simulink model "sst_cllc_ttype_inv"  (R2026a)
settings: Solver=ode23tb  StopTime=simlength  FixedStep=tc  MaxStep=glb_time.tc
values from neighbouring files (symbols this model uses):
  afe_ctrl = ctrl_afe_setup(glb_time.ts_afe, grid_emu.omega_grid_nom)    [init_model.m]
  cllc_ctrl = ctrl_cllc_setup(kp_udc, ki_udc, kp_idc, ki_idc)    [init_model.m]
  glb_time = timing_setup(fpwm_afe, trgo_afe, fpwm_inv, trgo_inv, fpwm_single_phase_inv, trgo_single_phase_inv, fpwm_dab, trgo_dab,      fpwm_psfbc, trgo_psfbc, fpwm_isop_rail, trgo_isop_rail, fpwm_cllc, trgo_cllc, t_measure, tc_factor, tc_decimation, delay_pwm, dead_time_afe,      dead_time_inv, dead_time_single_phase_inv, dead_time_dab, dead_time_psfbc, dead_time_isop_rail, dead_time_cllc)    [init_model.m]
  grid_emu = grid_three_phase_emulator('Dyn11', delta_star, grid_nominal_power, application_voltage, us1, us2, fgrid,                  eq_grid_inductance, eq_grid_resistance, eta, ucc, i1m, p_iron, n1, n2, core_area, core_length, mur,                  up_xi_pu_ref, up_eta_pu_ref, un_xi_pu_ref, un_eta_pu_ref)    [init_model.m]
  lithium_ion_battery_1 = lithium_ion_battery_setup(nominal_battery_voltage_1, nominal_battery_power, initial_battery_soc, glb_time.ts_dab)    [init_model.m]
  omega_set = frequency_set*2*pi    (= 1884.95559215)    [init_model.m]
  single_phase_inverter_ctrl = ctrl_single_phase_inverter_setup(glb_time.ts_inv, pres_ctrl.omega_set,      dqvector_pi.kp_inv, dqvector_pi.ki_inv, pres_ctrl.kp_rpi, pres_ctrl.ki_rpi, pres_ctrl.delta_rpi)    [init_model.m]
  sst_num_of_modules = 2    [init_model.m]
undefined symbols (not defined in the file or in its folder): hwdata
libraries: fl_lib x62, nesl_utility x38, discrete_time_low_pass_filter x8, full_bridge_ideal_switch x4, full_bridge_mosfet_based_with_thermal_model x4, full_bridge_mosfet_based_with_thermal_model_zvs x4, lithium_ion_battery x2, single_phase_transformer x2, dab_single_phase_pwm_modulator x2, dclink_for_three_levels x2, full_bridge_three_level_ttype_ideal_switch_based_model x2, full_bridge_three_level_ttype_mosfet_based_model x2
(part 2 of 5)

== system sst_cllc_ttype_inv/global timing/time_cllc_A ==
  correction_time : Inport
  Constant : Constant
  Gain : Gain  Gain=k
  Product : Product
  Sum : Sum  Inputs=|++
  time_1 : Clock
  Out1 : Outport
  wires:
  time_1/1 -> Gain/1
  Gain/1 -> Product/1
  Product/1 -> Out1/1
  correction_time/1 -> Sum/1
  Constant/1 -> Sum/2
  Sum/1 -> Product/2

== system sst_cllc_ttype_inv/global timing/time_cllc_B ==
  correction_time : Inport
  Constant : Constant
  Gain : Gain  Gain=k
  Product : Product
  Sum : Sum  Inputs=|++
  time_1 : Clock
  Out1 : Outport
  wires:
  time_1/1 -> Gain/1
  Gain/1 -> Product/1
  Product/1 -> Out1/1
  correction_time/1 -> Sum/1
  Constant/1 -> Sum/2
  Sum/1 -> Product/2

== system sst_cllc_ttype_inv/global timing/time_master ==
  Gain : Gain  Gain=k
  time_1 : Clock
  Out1 : Outport
  wires:
  Gain/1 -> Out1/1
  time_1/1 -> Gain/1

== system sst_cllc_ttype_inv/line_source/phase_gen ==
  Constant4 : Constant  Value=grid_emu.omega_grid_nom
  Integrator : Integrator
  bounder1 : MATLAB Function  TreatAsAtomicUnit=on
  phase_gen : Outport  VectorParamsAs1DForOutWhenUnconnected=off
  wires:
  Constant4/1 -> Integrator/1
  Integrator/1 -> bounder1/1(u)
  bounder1/1(y) -> phase_gen/1  "grid_emu_phase"

== system sst_cllc_ttype_inv/scopes/scopes_dcdc_modA ==
  Bus Selector : BusSelector  OutputSignals=mosfet_ploss_Q1,mosfet_ploss_Q2
  Bus Selector1 : BusSelector  OutputSignals=mosfet_ploss_Q1,mosfet_ploss_Q2
  cllc TR i2/i1 modA : Scope  NumInputPorts=2
      settings: ActiveDisplayYMinimum=-1515.8601129634949  ActiveDisplayYMaximum=1519.4045908602914  DataLoggingVariableName=ScopeData13
  cllc TR u2/u1 modA : Scope  NumInputPorts=2
      settings: ActiveDisplayYMinimum=-893.62031856834165  ActiveDisplayYMaximum=653.92363611228757  DataLoggingVariableName=ScopeData4
  cllc current output/input modA : Scope  NumInputPorts=2
      settings: ActiveDisplayYMinimum=-34.407086049322743  ActiveDisplayYMaximum=284.20809963586862  DataLoggingVariableName=ScopeData8
  cllc voltage input/output modA : Scope  NumInputPorts=2
      settings: ActiveDisplayYMinimum=-224.45374462345234  ActiveDisplayYMaximum=1977.0471198962268  DataLoggingVariableName=ScopeData10
  cllc_analysis_modA : Scope  NumInputPorts=4
      settings: ActiveDisplayYMinimum=-29.182723661894556  ActiveDisplayYMaximum=23.685544723854832  DataLoggingVariableName=ScopeData15
  cllc_analysis_power loss : Scope  NumInputPorts=4
      settings: ActiveDisplayYMinimum=17.348303631345402  ActiveDisplayYMaximum=238.28763733532384  DataLoggingVariableName=ScopeData17
  dab outputs modA : Scope  NumInputPorts=2
      settings: ActiveDisplayYMinimum=-691.31278967103344  ActiveDisplayYMaximum=557.00399497186572  DataLoggingVariableName=ScopeData6
  wires:
  [cllc_voltage_input_modA] -> cllc voltage input/output modA/1  "cllc_voltage_input_modA"
  [cllc_current_output_modA] -> cllc current output/input modA/1  "cllc_current_output_modA"
  [cllc_voltage_output_modA] -> cllc voltage input/output modA/2  "cllc_voltage_output_modA"
  [cllc_current_input_modA] -> cllc current output/input modA/2  "cllc_current_input_modA"
  [i2_cllc_transformer_modA] -> cllc TR i2/i1 modA/1  "i2_cllc_transformer_modA"
  [i1_cllc_transformer_modA] -> cllc TR i2/i1 modA/2  "i1_cllc_transformer_modA"
  [u2_cllc_transformer_modA] -> cllc TR u2/u1 modA/1  "u2_cllc_transformer_modA"
  [u1_cllc_transformer_modA] -> cllc TR u2/u1 modA/2  "u1_cllc_transformer_modA"
  [cllc_voltage_output_modA] -> dab outputs modA/2  "cllc_voltage_output_modA"
  [cllc_current_output_modA] -> dab outputs modA/1  "cllc_current_output_modA"
  [i2_cllc_transformer_modA] -> cllc_analysis_modA/1  "i2_cllc_transformer_modA"
  [i1_cllc_transformer_modA] -> cllc_analysis_modA/2  "i1_cllc_transformer_modA"
  [u1_cllc_transformer_modA] -> cllc_analysis_modA/3  "u1_cllc_transformer_modA"
  [u2_cllc_transformer_modA] -> cllc_analysis_modA/4  "u2_cllc_transformer_modA"
  [inverter_1_cllc_mosfet_zvs_modA] -> Bus Selector/1
  [inverter_2_cllc_mosfet_zvs_modA] -> Bus Selector1/1
  Bus Selector/1 -> cllc_analysis_power loss/1  "<mosfet_ploss_Q1>"
  Bus Selector/2 -> cllc_analysis_power loss/2  "<mosfet_ploss_Q2>"
  Bus Selector1/1 -> cllc_analysis_power loss/3  "<mosfet_ploss_Q1>"
  Bus Selector1/2 -> cllc_analysis_power loss/4  "<mosfet_ploss_Q2>"

== system sst_cllc_ttype_inv/scopes/scopes_dcdc_modB ==
  cllc TR i2/i1 modB : Scope  NumInputPorts=2
      settings: ActiveDisplayYMinimum=-700.08630880673149  ActiveDisplayYMaximum=469.74027472719069  DataLoggingVariableName=ScopeData13
  cllc TR u2/u1 modB : Scope  NumInputPorts=2
      settings: ActiveDisplayYMinimum=-893.62031856834165  ActiveDisplayYMaximum=653.92363611228757  DataLoggingVariableName=ScopeData4
  cllc current output/input modB : Scope  NumInputPorts=2
      settings: ActiveDisplayYMinimum=-7335.7913745283768  ActiveDisplayYMaximum=23819.434208451414  DataLoggingVariableName=ScopeData8
  cllc outputs modB : Scope  NumInputPorts=2
      settings: ActiveDisplayYMinimum=-1276.7812228163118  ActiveDisplayYMaximum=1202.3221787513703  DataLoggingVariableName=ScopeData6
  cllc voltage input/output modB : Scope  NumInputPorts=2
      settings: ActiveDisplayYMinimum=-237.60937353263552  ActiveDisplayYMaximum=2138.4843617937204  DataLoggingVariableName=ScopeData10
  cllc_analysis_modB : Scope  NumInputPorts=4
      settings: ActiveDisplayYMinimum=-1515.8601129634949  ActiveDisplayYMaximum=1519.4045908602914  DataLoggingVariableName=ScopeData15
  wires:
  [u2_cllc_transformer_modB] -> cllc_analysis_modB/4  "u2_cllc_transformer_modB"
  [u1_cllc_transformer_modB] -> cllc_analysis_modB/3  "u1_cllc_transformer_modB"
  [i1_cllc_transformer_modB] -> cllc_analysis_modB/2  "i1_cllc_transformer_modB"
  [i2_cllc_transformer_modB] -> cllc_analysis_modB/1  "i2_cllc_transformer_modB"
  [cllc_current_output_modB] -> cllc outputs modB/1  "cllc_current_output_modB"
  [cllc_voltage_output_modB] -> cllc outputs modB/2  "cllc_voltage_output_modB"
  [u1_cllc_transformer_modB] -> cllc TR u2/u1 modB/2  "u1_cllc_transformer_modB"
  [u2_cllc_transformer_modB] -> cllc TR u2/u1 modB/1  "u2_cllc_transformer_modB"
  [i1_cllc_transformer_modB] -> cllc TR i2/i1 modB/2  "i1_cllcb_transformer_modB"
  [i2_cllc_transformer_modB] -> cllc TR i2/i1 modB/1  "i2_cllc_transformer_modB"
  [cllc_current_input_modB] -> cllc current output/input modB/2  "cllc_current_input_modB"
  [cllc_voltage_output_modB] -> cllc voltage input/output modB/2  "cllc_voltage_output_modB"
  [cllc_current_output_modB] -> cllc current output/input modB/1  "cllc_current_output_modB"
  [cllc_voltage_input_modB] -> cllc voltage input/output modB/1  "cllc_voltage_input_modB"

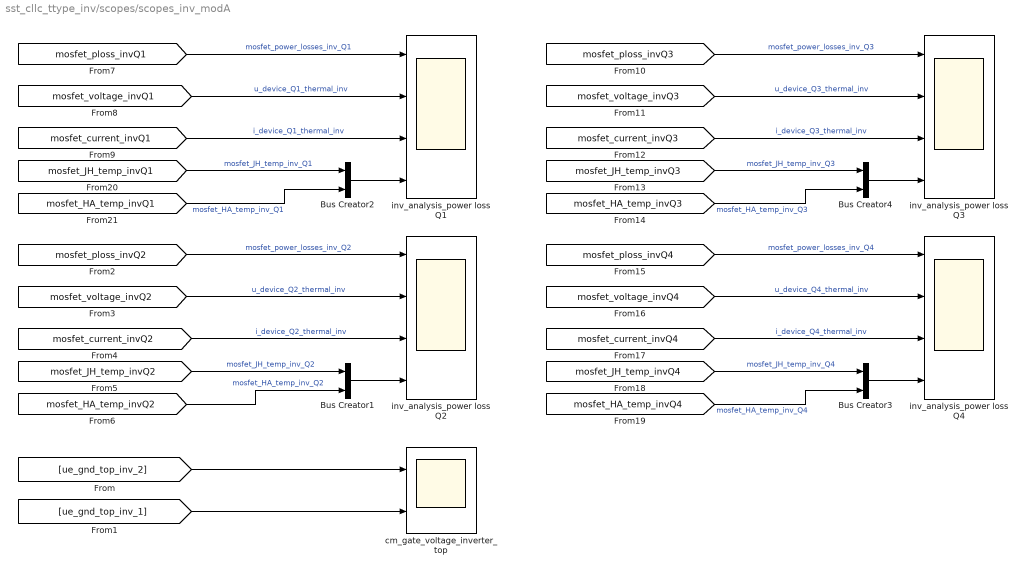
== system sst_cllc_ttype_inv/scopes/scopes_inv_modA ==
  Bus Creator{1..4} (4 alike) : BusCreator  Inputs=2
  cm_gate_voltage_inverter_top : Scope  NumInputPorts=2
      settings: ActiveDisplayYMinimum=-1089.6954299405313  ActiveDisplayYMaximum=1165.8713445946826  DataLoggingVariableName=ScopeData22
  inv_analysis_power loss Q{1..4} (4 alike) : Scope  NumInputPorts=4
      inv_analysis_power loss Q1 settings: ActiveDisplayYMinimum=252.03887543128099  ActiveDisplayYMaximum=654.5130246681365  DataLoggingVariableName=ScopeData18
      inv_analysis_power loss Q2 settings: ActiveDisplayYMinimum=1215.5585157804567  ActiveDisplayYMaximum=1882.3509853926439  DataLoggingVariableName=ScopeData5
      inv_analysis_power loss Q3 settings: ActiveDisplayYMinimum=1399.7218598743666  ActiveDisplayYMaximum=1614.3940109339064  DataLoggingVariableName=ScopeData16
      inv_analysis_power loss Q4 settings: ActiveDisplayYMinimum=401.80036733196005  ActiveDisplayYMaximum=489.90080295034829  DataLoggingVariableName=ScopeData19
  wires:
  [mosfet_JH_temp_invQ1] -> Bus Creator2/1  "mosfet_JH_temp_inv_Q1"
  [mosfet_voltage_invQ1] -> inv_analysis_power loss Q1/2  "u_device_Q1_thermal_inv"
  [mosfet_current_invQ1] -> inv_analysis_power loss Q1/3  "i_device_Q1_thermal_inv"
  [mosfet_HA_temp_invQ1] -> Bus Creator2/2  "mosfet_HA_temp_inv_Q1"
  Bus Creator2/1 -> inv_analysis_power loss Q1/4
  [mosfet_ploss_invQ1] -> inv_analysis_power loss Q1/1  "mosfet_power_losses_inv_Q1"
  [ue_gnd_top_inv_2] -> cm_gate_voltage_inverter_top/1
  [ue_gnd_top_inv_1] -> cm_gate_voltage_inverter_top/2
  [mosfet_ploss_invQ2] -> inv_analysis_power loss Q2/1  "mosfet_power_losses_inv_Q2"
  Bus Creator1/1 -> inv_analysis_power loss Q2/4
  [mosfet_HA_temp_invQ2] -> Bus Creator1/2  "mosfet_HA_temp_inv_Q2"
  [mosfet_current_invQ2] -> inv_analysis_power loss Q2/3  "i_device_Q2_thermal_inv"
  [mosfet_voltage_invQ2] -> inv_analysis_power loss Q2/2  "u_device_Q2_thermal_inv"
  [mosfet_JH_temp_invQ2] -> Bus Creator1/1  "mosfet_JH_temp_inv_Q2"
  [mosfet_JH_temp_invQ4] -> Bus Creator3/1  "mosfet_JH_temp_inv_Q4"
  [mosfet_voltage_invQ4] -> inv_analysis_power loss Q4/2  "u_device_Q4_thermal_inv"
  [mosfet_current_invQ4] -> inv_analysis_power loss Q4/3  "i_device_Q4_thermal_inv"
  [mosfet_HA_temp_invQ4] -> Bus Creator3/2  "mosfet_HA_temp_inv_Q4"
  Bus Creator3/1 -> inv_analysis_power loss Q4/4
  [mosfet_ploss_invQ4] -> inv_analysis_power loss Q4/1  "mosfet_power_losses_inv_Q4"
  [mosfet_ploss_invQ3] -> inv_analysis_power loss Q3/1  "mosfet_power_losses_inv_Q3"
  Bus Creator4/1 -> inv_analysis_power loss Q3/4
  [mosfet_HA_temp_invQ3] -> Bus Creator4/2  "mosfet_HA_temp_inv_Q3"
  [mosfet_current_invQ3] -> inv_analysis_power loss Q3/3  "i_device_Q3_thermal_inv"
  [mosfet_voltage_invQ3] -> inv_analysis_power loss Q3/2  "u_device_Q3_thermal_inv"
  [mosfet_JH_temp_invQ3] -> Bus Creator4/1  "mosfet_JH_temp_inv_Q3"

== system sst_cllc_ttype_inv/scopes/scopes_inv_modB ==
  cm_gate_voltage_inverter_bottom : Scope  NumInputPorts=2
      settings: ActiveDisplayYMinimum=-1241.6958905586757  ActiveDisplayYMaximum=1224.9152234663466  DataLoggingVariableName=ScopeData22
  device_voltage_current_inv Q1 modB : Scope  NumInputPorts=3
      settings: ActiveDisplayYMinimum=-119.06518095025848  ActiveDisplayYMaximum=1054.0032225267662  DataLoggingVariableName=ScopeData20
  wires:
  [ue_gnd_bottom_inv_1] -> cm_gate_voltage_inverter_bottom/2
  [ue_gnd_bottom_inv_2] -> cm_gate_voltage_inverter_bottom/1
  [i_device_Q1_ideal_inv_modB] -> device_voltage_current_inv Q1 modB/2  "iQ1"
  [u_device_Q1_ideal_inv_modB] -> device_voltage_current_inv Q1 modB/1  "uQ1"
  [udc12_inverter_modB] -> device_voltage_current_inv Q1 modB/3  "udcs"

== system sst_cllc_ttype_inv/single_phase_inverter_modA/dclink ==
  Open Circuit : fl_lib/Electrical/Electrical Elements/Open Circuit  v_specify=off  v_priority=None  v=0 V  v_nominal_specify=off  v_nominal_value=1  v_nominal_unit=V
  dclink : dclink_for_three_levels/dclink  Cdc1_m=hwdata.single_phase_inverter.CFi1  Cdc2_m=hwdata.single_phase_inverter.CFi2  Rudc_measure=107e3  Vdc_scale=hwdata.cllc.udc2_bez  Vdc1_m_init=hwdata.cllc.udc2_bez/2  Vdc2_m_init=hwdata.cllc.udc2_bez/2
  references : Subsystem
  Udc(+) : PMIOPort  Side=Right
  np : PMIOPort  Port=2  Side=Right
  Udc(-) : PMIOPort  Port=3  Side=Right
  udc(+) : PMIOPort  Port=4  Side=Left
  udc(-) : PMIOPort  Port=5  Side=Left
  wires:
  dclink/1 -> references/1(m)
  connections:
  Open Circuit/LConn1 -- dclink/RConn2
  udc(+)/RConn1 -- dclink/RConn1
  udc(-)/RConn1 -- dclink/RConn3
  Udc(+)/RConn1 -- dclink/LConn1
  Udc(-)/RConn1 -- dclink/LConn3
  dclink/LConn2 -- np/RConn1

== system sst_cllc_ttype_inv/single_phase_inverter_modA/output_filter ==
  Capacitor : fl_lib/Electrical/Electrical Elements/Capacitor  c=hwdata.single_phase_inverter.CFu F  r=hwdata.single_phase_inverter.RCFu Ohm  g=0 1/Ohm  i_specify=off  i_priority=None  i=0 A  i_nominal_specify=off  i_nominal_value=1  i_nominal_unit=A  v_specify=off  v_priority=None  v=0 V  v_nominal_specify=off  v_nominal_value=1  v_nominal_unit=V  vc_specify=off  vc_priority=High  vc=0 V  vc_nominal_specify=off  vc_nominal_value=1  vc_nominal_unit=V
  Current Sensor : fl_lib/Electrical/Electrical Sensors/Current Sensor
  Current Sensor1 : fl_lib/Electrical/Electrical Sensors/Current Sensor
  LFu1 : fl_lib/Electrical/Electrical Elements/Inductor  l=hwdata.single_phase_inverter.LFu1 H  r=hwdata.single_phase_inverter.RLFu1 Ohm  g=1e-9 1/Ohm  i_specify=off  i_priority=None  i=0 A  i_nominal_specify=off  i_nominal_value=1  i_nominal_unit=A  v_specify=off  v_priority=None  v=0 V  v_nominal_specify=off  v_nominal_value=1  v_nominal_unit=V  i_L_specify=off  i_L_priority=High  i_L=0 A  i_L_nominal_specify=off  i_L_nominal_value=1  i_L_nominal_unit=A
  LFu2 : fl_lib/Electrical/Electrical Elements/Inductor  l=hwdata.single_phase_inverter.LFu2 H  r=hwdata.single_phase_inverter.RLFu2 Ohm  g=1e-9 1/Ohm  i_specify=off  i_priority=None  i=0 A  i_nominal_specify=off  i_nominal_value=1  i_nominal_unit=A  v_specify=off  v_priority=None  v=0 V  v_nominal_specify=off  v_nominal_value=1  v_nominal_unit=V  i_L_specify=off  i_L_priority=High  i_L=0 A  i_L_nominal_specify=off  i_L_nominal_value=1  i_L_nominal_unit=A
  Voltage Sensor1 : fl_lib/Electrical/Electrical Sensors/Voltage Sensor
  Voltage Sensor2 : fl_lib/Electrical/Electrical Sensors/Voltage Sensor
  iph : nesl_utility/PS-Simulink Converter  PhysicalDomain=network_engine_domain  SubClassName=ps_output  LeftPortType=input  RightPortType=output  PseudoPeriodic=off  Frequencies=[]  VectorFormat=1-D array  Unit=A  AffineConversion=off
  iph1 : nesl_utility/PS-Simulink Converter  PhysicalDomain=network_engine_domain  SubClassName=ps_output  LeftPortType=input  RightPortType=output  PseudoPeriodic=off  Frequencies=[]  VectorFormat=1-D array  Unit=A  AffineConversion=off
  uph1 : nesl_utility/PS-Simulink Converter  PhysicalDomain=network_engine_domain  SubClassName=ps_output  LeftPortType=input  RightPortType=output  PseudoPeriodic=off  Frequencies=[]  VectorFormat=1-D array  Unit=V  AffineConversion=off
  uph2 : nesl_utility/PS-Simulink Converter  PhysicalDomain=network_engine_domain  SubClassName=ps_output  LeftPortType=input  RightPortType=output  PseudoPeriodic=off  Frequencies=[]  VectorFormat=1-D array  Unit=V  AffineConversion=off
  Uac(+) : PMIOPort  Side=Left
  uac(+) : PMIOPort  Port=2  Side=Right
  Uac(-) : PMIOPort  Port=3  Side=Left
  uac(-) : PMIOPort  Port=4  Side=Right
  tag scope: afe_current_output_modA=global, afe_is_modA=global, afe_us_modA=global, afe_voltage_output_modA=global
  wires:
  uph1/1 -> [afe_voltage_output_modA]  "inverter_voltage_output"
  iph/1 -> [afe_current_output_modA]  "inverter_current_output"
  iph1/1 -> [afe_is_modA]  "inverter_is_modA"
  uph2/1 -> [afe_us_modA]  "inverter_us_modA"
  connections:
  Voltage Sensor2/LConn1 -- Current Sensor1/RConn2 -- LFu1/LConn1
  Current Sensor/RConn2 -- uac(+)/RConn1 -- Voltage Sensor1/LConn1
  Voltage Sensor1/RConn2 -- Capacitor/RConn1 -- LFu2/RConn1 -- uac(-)/RConn1
  iph/LConn1 -- Current Sensor/RConn1
  Voltage Sensor1/RConn1 -- uph1/LConn1
  LFu1/RConn1 -- Capacitor/LConn1 -- Current Sensor/LConn1
  Uac(-)/RConn1 -- Voltage Sensor2/RConn2 -- LFu2/LConn1
  iph1/LConn1 -- Current Sensor1/RConn1
  Voltage Sensor2/RConn1 -- uph2/LConn1
  Uac(+)/RConn1 -- Current Sensor1/LConn1

== system sst_cllc_ttype_inv/single_phase_inverter_modA/single phase afe ==
  gate_commands : Inport
  ideal_switch_based_three_level_inverter_ttype : full_bridge_three_level_ttype_ideal_switch_based_model/ideal_switch_based_three_level_inverter_ttype  Commented=on  Vth=ideal_switch.Vth  Ron=ideal_switch.Rds_on  Vdon_diode=ideal_switch.Vdon_diode  Rdon_diode=ideal_switch.Rdon_diode  Csnubber=ideal_switch.Csnubber  Rsnubber=ideal_switch.Rsnubber
  mosfet_based_three_level_inverter_ttype : full_bridge_three_level_ttype_mosfet_based_model/mosfet_based_three_level_inverter_ttype  Vth_m=mosfet.inv.Vth  Rds_on_m=mosfet.inv.Rds_on  Eon_m=mosfet.inv.Eon  Eoff_m=mosfet.inv.Eoff  Erec_m=mosfet.inv.Err  Ion_sw_loss_m=mosfet.inv.Ion_sw_losses  Voff_sw_loss_m=mosfet.inv.Voff_sw_losses  Vdon_diode_m=mosfet.inv.Vdon_diode  Rdon_diode_m=mosfet.inv.Rdon_diode  rth_mosfet_JH_m=mosfet.inv.Rth_mosfet_JH  rth_mosfet_HA_m=heatsink.Rth_mosfet_HA  Csnubber_m=mosfet.inv.Csnubber  Rsnubber_m=mosfet.inv.Rsnubber  JunctionTermalMass_m=mosfet.inv.JunctionTermalMass  mass_heatsink_m=heatsink.no_weight  specific_heat_m=heatsink.cp  Tambient_m=heatsink.Tambient  DThs_init_m=heatsink.DThs_init  tc_m=glb_time.tc
  references : Subsystem
  uac_out(+) : PMIOPort  Side=Left
  uac_out(-) : PMIOPort  Port=2  Side=Left
  udc(+) : PMIOPort  Port=3  Side=Right
  np : PMIOPort  Port=4  Side=Right
  udc(-) : PMIOPort  Port=5  Side=Right
  wires:
  gate_commands/1 -> mosfet_based_three_level_inverter_ttype/1, ideal_switch_based_three_level_inverter_ttype/1
  mosfet_based_three_level_inverter_ttype/1 -> references/1(m)
  connections:
  ideal_switch_based_three_level_inverter_ttype/LConn2 -- mosfet_based_three_level_inverter_ttype/LConn2 -- uac_out(-)/RConn1
  ideal_switch_based_three_level_inverter_ttype/RConn1 -- mosfet_based_three_level_inverter_ttype/RConn1 -- udc(+)/RConn1
  ideal_switch_based_three_level_inverter_ttype/LConn1 -- mosfet_based_three_level_inverter_ttype/LConn1 -- uac_out(+)/RConn1
  ideal_switch_based_three_level_inverter_ttype/RConn3 -- mosfet_based_three_level_inverter_ttype/RConn3 -- udc(-)/RConn1
  ideal_switch_based_three_level_inverter_ttype/RConn2 -- mosfet_based_three_level_inverter_ttype/RConn2 -- np/RConn1

== system sst_cllc_ttype_inv/single_phase_inverter_modA/single phase inverter control ==
  acquisition_and_scaling_current : Subsystem  Commented=on
  acquisition_and_scaling_current_with_white_noise : Subsystem
  acquisition_and_scaling_dc_voltage : Subsystem
  acquisition_and_scaling_grid_voltage_ac : Subsystem
  acquisition_and_scaling_voltage : Subsystem
  inverter_current_output_pu_reference : Subsystem
  pwm modulator : Subsystem
  single_phase_inverter_ctrl : Subsystem
  gate_cmds : Outport
  tag scope: afe_phase_grid_hat_modA=global, udq_ctrl_out_modA=global
  wires:
  [afe_is_modA] -> acquisition_and_scaling_current_with_white_noise/1(in)
  pwm modulator/1(gate_cmds) -> gate_cmds/1
  [TRGO_AFE_modA] -> single_phase_inverter_ctrl/Trigger
  [afe_voltage_output_modA] -> acquisition_and_scaling_voltage/1(in)
  single_phase_inverter_ctrl/1(u_ctrl_out) -> pwm modulator/1(vout)
  acquisition_and_scaling_current_with_white_noise/1(out) -> single_phase_inverter_ctrl/2(afe_current_output_pu)  "afe_current_output_pu"
  acquisition_and_scaling_voltage/1(out) -> single_phase_inverter_ctrl/1(afe_voltage_output_pu)  "afe_voltage_output_pu"
  inverter_current_output_pu_reference/1(afe_current_output_pu_reference) -> single_phase_inverter_ctrl/3(afe_current output_pu_reference)  "afe_current_output_pu_reference"
  [dclink_voltage_modA] -> acquisition_and_scaling_dc_voltage/1(in)
  acquisition_and_scaling_dc_voltage/1(out) -> single_phase_inverter_ctrl/4(dclink_voltage_pu)  "dclink_voltage_pu"
  [time_afe_module_A] -> single_phase_inverter_ctrl/5(local_time)
  [ac_grid_voltage] -> acquisition_and_scaling_grid_voltage_ac/1(in)
  acquisition_and_scaling_grid_voltage_ac/1(out) -> single_phase_inverter_ctrl/6(ugrid_pu)  "ug_abc"
  single_phase_inverter_ctrl/2(phase_grid_hat) -> [afe_phase_grid_hat_modA]
  single_phase_inverter_ctrl/3(udq_ctrl_out) -> [udq_ctrl_out_modA]

== system sst_cllc_ttype_inv/single_phase_inverter_modB/dclink ==
  Open Circuit : fl_lib/Electrical/Electrical Elements/Open Circuit  v_specify=off  v_priority=None  v=0 V  v_nominal_specify=off  v_nominal_value=1  v_nominal_unit=V
  dclink : dclink_for_three_levels/dclink  Cdc1_m=hwdata.single_phase_inverter.CFi1  Cdc2_m=hwdata.single_phase_inverter.CFi2  Rudc_measure=107e3  Vdc_scale=hwdata.cllc.udc2_bez  Vdc1_m_init=hwdata.cllc.udc2_bez/2  Vdc2_m_init=hwdata.cllc.udc2_bez/2
  references : Subsystem
  Udc(+) : PMIOPort  Side=Right
  np : PMIOPort  Port=2  Side=Right
  Udc(-) : PMIOPort  Port=3  Side=Right
  udc(+) : PMIOPort  Port=4  Side=Left
  udc(-) : PMIOPort  Port=5  Side=Left
  wires:
  dclink/1 -> references/1(m)
  connections:
  dclink/LConn2 -- np/RConn1
  Udc(-)/RConn1 -- dclink/LConn3
  Udc(+)/RConn1 -- dclink/LConn1
  udc(-)/RConn1 -- dclink/RConn3
  udc(+)/RConn1 -- dclink/RConn1
  Open Circuit/LConn1 -- dclink/RConn2

== system sst_cllc_ttype_inv/single_phase_inverter_modB/output_filter ==
  Capacitor : fl_lib/Electrical/Electrical Elements/Capacitor  c=hwdata.single_phase_inverter.CFu F  r=hwdata.single_phase_inverter.RCFu Ohm  g=0 1/Ohm  i_specify=off  i_priority=None  i=0 A  i_nominal_specify=off  i_nominal_value=1  i_nominal_unit=A  v_specify=off  v_priority=None  v=0 V  v_nominal_specify=off  v_nominal_value=1  v_nominal_unit=V  vc_specify=off  vc_priority=High  vc=0 V  vc_nominal_specify=off  vc_nominal_value=1  vc_nominal_unit=V
  Current Sensor : fl_lib/Electrical/Electrical Sensors/Current Sensor
  Current Sensor1 : fl_lib/Electrical/Electrical Sensors/Current Sensor
  LFu1 : fl_lib/Electrical/Electrical Elements/Inductor  l=hwdata.single_phase_inverter.LFu1 H  r=hwdata.single_phase_inverter.RLFu1 Ohm  g=1e-9 1/Ohm  i_specify=off  i_priority=None  i=0 A  i_nominal_specify=off  i_nominal_value=1  i_nominal_unit=A  v_specify=off  v_priority=None  v=0 V  v_nominal_specify=off  v_nominal_value=1  v_nominal_unit=V  i_L_specify=off  i_L_priority=High  i_L=0 A  i_L_nominal_specify=off  i_L_nominal_value=1  i_L_nominal_unit=A
  LFu2 : fl_lib/Electrical/Electrical Elements/Inductor  l=hwdata.single_phase_inverter.LFu2 H  r=hwdata.single_phase_inverter.RLFu2 Ohm  g=1e-9 1/Ohm  i_specify=off  i_priority=None  i=0 A  i_nominal_specify=off  i_nominal_value=1  i_nominal_unit=A  v_specify=off  v_priority=None  v=0 V  v_nominal_specify=off  v_nominal_value=1  v_nominal_unit=V  i_L_specify=off  i_L_priority=High  i_L=0 A  i_L_nominal_specify=off  i_L_nominal_value=1  i_L_nominal_unit=A
  Voltage Sensor1 : fl_lib/Electrical/Electrical Sensors/Voltage Sensor
  Voltage Sensor2 : fl_lib/Electrical/Electrical Sensors/Voltage Sensor
  iph : nesl_utility/PS-Simulink Converter  PhysicalDomain=network_engine_domain  SubClassName=ps_output  LeftPortType=input  RightPortType=output  PseudoPeriodic=off  Frequencies=[]  VectorFormat=1-D array  Unit=A  AffineConversion=off
  iph1 : nesl_utility/PS-Simulink Converter  PhysicalDomain=network_engine_domain  SubClassName=ps_output  LeftPortType=input  RightPortType=output  PseudoPeriodic=off  Frequencies=[]  VectorFormat=1-D array  Unit=A  AffineConversion=off
  uph1 : nesl_utility/PS-Simulink Converter  PhysicalDomain=network_engine_domain  SubClassName=ps_output  LeftPortType=input  RightPortType=output  PseudoPeriodic=off  Frequencies=[]  VectorFormat=1-D array  Unit=V  AffineConversion=off
  uph2 : nesl_utility/PS-Simulink Converter  PhysicalDomain=network_engine_domain  SubClassName=ps_output  LeftPortType=input  RightPortType=output  PseudoPeriodic=off  Frequencies=[]  VectorFormat=1-D array  Unit=V  AffineConversion=off
  Uac(+) : PMIOPort  Side=Left
  uac(+) : PMIOPort  Port=2  Side=Right
  Uac(-) : PMIOPort  Port=3  Side=Left
  uac(-) : PMIOPort  Port=4  Side=Right
  tag scope: afe_current_output_modB=global, afe_is_modB=global, afe_us_modB=global, afe_voltage_output_modB=global
  wires:
  uph2/1 -> [afe_us_modB]  "inverter_us_modA"
  iph1/1 -> [afe_is_modB]  "inverter_is_modA"
  iph/1 -> [afe_current_output_modB]  "inverter_current_output"
  uph1/1 -> [afe_voltage_output_modB]  "inverter_voltage_output"
  connections:
  Uac(+)/RConn1 -- Current Sensor1/LConn1
  Voltage Sensor2/RConn1 -- uph2/LConn1
  iph1/LConn1 -- Current Sensor1/RConn1
  LFu2/LConn1 -- Voltage Sensor2/RConn2 -- Uac(-)/RConn1
  Current Sensor/LConn1 -- Capacitor/LConn1 -- LFu1/RConn1
  Voltage Sensor1/RConn1 -- uph1/LConn1
  iph/LConn1 -- Current Sensor/RConn1
  uac(-)/RConn1 -- LFu2/RConn1 -- Capacitor/RConn1 -- Voltage Sensor1/RConn2
  Voltage Sensor1/LConn1 -- uac(+)/RConn1 -- Current Sensor/RConn2
  LFu1/LConn1 -- Current Sensor1/RConn2 -- Voltage Sensor2/LConn1

== system sst_cllc_ttype_inv/single_phase_inverter_modB/single phase afe ==
  gate_commands : Inport
  ideal_switch_based_three_level_inverter_ttype : full_bridge_three_level_ttype_ideal_switch_based_model/ideal_switch_based_three_level_inverter_ttype  Vth=ideal_switch.Vth  Ron=ideal_switch.Rds_on  Vdon_diode=ideal_switch.Vdon_diode  Rdon_diode=ideal_switch.Rdon_diode  Csnubber=ideal_switch.Csnubber  Rsnubber=ideal_switch.Rsnubber
  mosfet_based_three_level_inverter_ttype : full_bridge_three_level_ttype_mosfet_based_model/mosfet_based_three_level_inverter_ttype  Commented=on  Vth_m=mosfet.inv.Vth  Rds_on_m=mosfet.inv.Rds_on  Eon_m=mosfet.inv.Eon  Eoff_m=mosfet.inv.Eoff  Erec_m=mosfet.inv.Err  Ion_sw_loss_m=mosfet.inv.Ion_sw_losses  Voff_sw_loss_m=mosfet.inv.Voff_sw_losses  Vdon_diode_m=mosfet.inv.Vdon_diode  Rdon_diode_m=mosfet.inv.Rdon_diode  rth_mosfet_JH_m=mosfet.inv.Rth_mosfet_JH  rth_mosfet_HA_m=heatsink.Rth_mosfet_HA  Csnubber_m=mosfet.inv.Csnubber  Rsnubber_m=mosfet.inv.Rsnubber  JunctionTermalMass_m=mosfet.inv.JunctionTermalMass  mass_heatsink_m=heatsink.no_weight  specific_heat_m=heatsink.cp  Tambient_m=heatsink.Tambient  DThs_init_m=heatsink.DThs_init  tc_m=glb_time.tc
  references : Subsystem  Commented=on
  uac_out(+) : PMIOPort  Side=Left
  uac_out(-) : PMIOPort  Port=2  Side=Left
  udc(+) : PMIOPort  Port=3  Side=Right
  np : PMIOPort  Port=4  Side=Right
  udc(-) : PMIOPort  Port=5  Side=Right
  wires:
  mosfet_based_three_level_inverter_ttype/1 -> references/1(m)
  gate_commands/1 -> ideal_switch_based_three_level_inverter_ttype/1, mosfet_based_three_level_inverter_ttype/1
  connections:
  np/RConn1 -- mosfet_based_three_level_inverter_ttype/RConn2 -- ideal_switch_based_three_level_inverter_ttype/RConn2
  udc(-)/RConn1 -- mosfet_based_three_level_inverter_ttype/RConn3 -- ideal_switch_based_three_level_inverter_ttype/RConn3
  uac_out(+)/RConn1 -- mosfet_based_three_level_inverter_ttype/LConn1 -- ideal_switch_based_three_level_inverter_ttype/LConn1
  udc(+)/RConn1 -- mosfet_based_three_level_inverter_ttype/RConn1 -- ideal_switch_based_three_level_inverter_ttype/RConn1
  uac_out(-)/RConn1 -- mosfet_based_three_level_inverter_ttype/LConn2 -- ideal_switch_based_three_level_inverter_ttype/LConn2

== system sst_cllc_ttype_inv/single_phase_inverter_modB/single phase inverter control ==
  acquisition_and_scaling_current_with_white_noise : Subsystem
  acquisition_and_scaling_dc_voltage : Subsystem
  acquisition_and_scaling_grid_voltage_ac : Subsystem
  acquisition_and_scaling_voltage : Subsystem
  inverter_current_output_pu_reference : Subsystem
  pwm modulator : Subsystem
  single_phase_inverter_ctrl : Subsystem
  gate_cmds : Outport
  tag scope: afe_phase_grid_hat_modB=global
  wires:
  single_phase_inverter_ctrl/2(phase_grid_hat) -> [afe_phase_grid_hat_modB]
  acquisition_and_scaling_grid_voltage_ac/1(out) -> single_phase_inverter_ctrl/6(ugrid_pu)  "ug_abc"
  [ac_grid_voltage] -> acquisition_and_scaling_grid_voltage_ac/1(in)
  [time_afe_module_B] -> single_phase_inverter_ctrl/5(local_time)
  acquisition_and_scaling_dc_voltage/1(out) -> single_phase_inverter_ctrl/4(dclink_voltage_pu)  "dclink_voltage_pu"
  [dclink_voltage_modB] -> acquisition_and_scaling_dc_voltage/1(in)
  inverter_current_output_pu_reference/1(afe_current_output_pu_reference) -> single_phase_inverter_ctrl/3(afe_current output_pu_reference)  "afe_current_output_pu_reference"
  acquisition_and_scaling_voltage/1(out) -> single_phase_inverter_ctrl/1(afe_voltage_output_pu)  "afe_voltage_output_pu"
  acquisition_and_scaling_current_with_white_noise/1(out) -> single_phase_inverter_ctrl/2(afe_current_output_pu)  "afe_current_output_pu"
  single_phase_inverter_ctrl/1(u_ctrl_out) -> pwm modulator/1(vout)
  [afe_voltage_output_modB] -> acquisition_and_scaling_voltage/1(in)
  [TRGO_AFE_modB] -> single_phase_inverter_ctrl/Trigger
  pwm modulator/1(gate_cmds) -> gate_cmds/1
  [afe_is_modB] -> acquisition_and_scaling_current_with_white_noise/1(in)
  [udq_ctrl_out_modA] -> single_phase_inverter_ctrl/7(udq_ctrl_out)

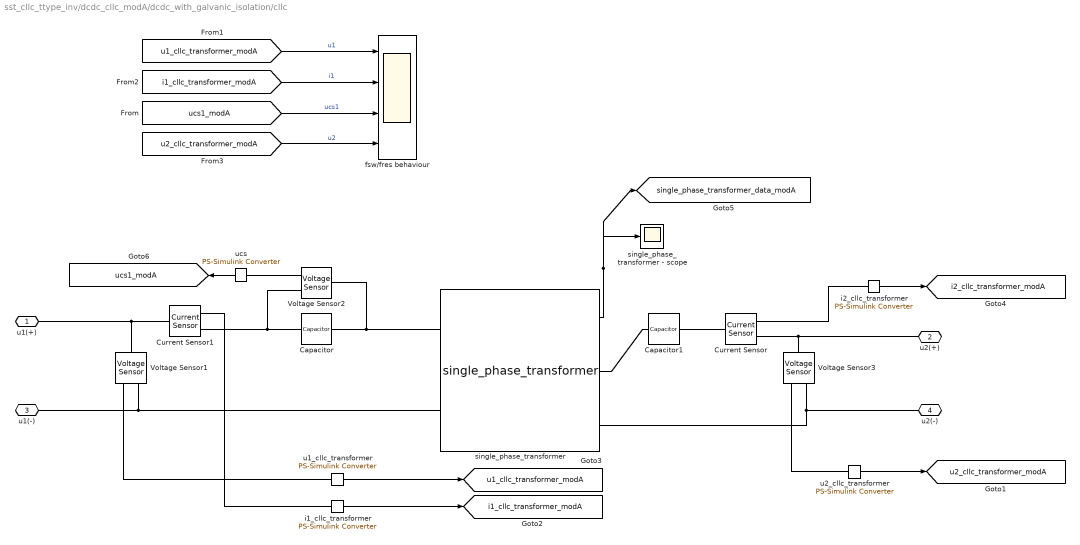
== system sst_cllc_ttype_inv/dcdc_cllc_modA/dcdc_with_galvanic_isolation/cllc ==
  Capacitor : fl_lib/Electrical/Electrical Elements/Capacitor  c=hwdata.cllc.Cs1 F  r=1e-6 Ohm  g=0 1/Ohm  i_specify=off  i_priority=None  i=0 A  i_nominal_specify=off  i_nominal_value=1  i_nominal_unit=A  v_specify=off  v_priority=None  v=0 V  v_nominal_specify=off  v_nominal_value=1  v_nominal_unit=V  vc_specify=off  vc_priority=High  vc=0 V  vc_nominal_specify=off  vc_nominal_value=1  vc_nominal_unit=V
  Capacitor1 : fl_lib/Electrical/Electrical Elements/Capacitor  c=hwdata.cllc.Cs2 F  r=1e-6 Ohm  g=0 1/Ohm  i_specify=off  i_priority=None  i=0 A  i_nominal_specify=off  i_nominal_value=1  i_nominal_unit=A  v_specify=off  v_priority=None  v=0 V  v_nominal_specify=off  v_nominal_value=1  v_nominal_unit=V  vc_specify=off  vc_priority=High  vc=0 V  vc_nominal_specify=off  vc_nominal_value=1  vc_nominal_unit=V
  Current Sensor : fl_lib/Electrical/Electrical Sensors/Current Sensor
  Current Sensor1 : fl_lib/Electrical/Electrical Sensors/Current Sensor
  Voltage Sensor1 : fl_lib/Electrical/Electrical Sensors/Voltage Sensor
  Voltage Sensor2 : fl_lib/Electrical/Electrical Sensors/Voltage Sensor
  Voltage Sensor3 : fl_lib/Electrical/Electrical Sensors/Voltage Sensor
  fsw/fres behaviour : Scope  NumInputPorts=4
      settings: ActiveDisplayYMinimum=-4267.1609835025592  ActiveDisplayYMaximum=3383.5844318464588  DataLoggingVariableName=ScopeData14
  i1_cllc_transformer : nesl_utility/PS-Simulink Converter  PhysicalDomain=network_engine_domain  SubClassName=ps_output  LeftPortType=input  RightPortType=output  PseudoPeriodic=off  Frequencies=[]  VectorFormat=1-D array  Unit=A  AffineConversion=off
  i2_cllc_transformer : nesl_utility/PS-Simulink Converter  PhysicalDomain=network_engine_domain  SubClassName=ps_output  LeftPortType=input  RightPortType=output  PseudoPeriodic=off  Frequencies=[]  VectorFormat=1-D array  Unit=A  AffineConversion=off
  single_phase_transformer : single_phase_transformer/single_phase_transformer  lm_trafo=hwdata.cllc.Lm  m1=hwdata.cllc.n1  m2=hwdata.cllc.n2  rd1_trafo=hwdata.cllc.Rs1  rd2_trafo=hwdata.cllc.Rs2  ld1_trafo=hwdata.cllc.Ld1  ld2_trafo=hwdata.cllc.Ld2  rfe_trafo=hwdata.cllc.Rfe  length_core=hwdata.cllc.core_length  mu0=1.256637e-6  mur=hwdata.cllc.core_mur
  single_phase_transformer - scope : Scope
      settings: ActiveDisplayYMinimum=-6684.1656967268027  ActiveDisplayYMaximum=6541.9063556817082  DataLoggingVariableName=ScopeData21
  u1_cllc_transformer : nesl_utility/PS-Simulink Converter  PhysicalDomain=network_engine_domain  SubClassName=ps_output  LeftPortType=input  RightPortType=output  PseudoPeriodic=off  Frequencies=[]  VectorFormat=1-D array  Unit=V  AffineConversion=on
  u2_cllc_transformer : nesl_utility/PS-Simulink Converter  PhysicalDomain=network_engine_domain  SubClassName=ps_output  LeftPortType=input  RightPortType=output  PseudoPeriodic=off  Frequencies=[]  VectorFormat=1-D array  Unit=V  AffineConversion=on
  ucs : nesl_utility/PS-Simulink Converter  PhysicalDomain=network_engine_domain  SubClassName=ps_output  LeftPortType=input  RightPortType=output  PseudoPeriodic=off  Frequencies=[]  VectorFormat=1-D array  Unit=V  AffineConversion=on
  u1(+) : PMIOPort  Side=Left
  u2(+) : PMIOPort  Port=2  Side=Right
  u1(-) : PMIOPort  Port=3  Side=Left
  u2(-) : PMIOPort  Port=4  Side=Right
  tag scope: i1_cllc_transformer_modA=global, i2_cllc_transformer_modA=global, single_phase_transformer_data_modA=global, u1_cllc_transformer_modA=global, u2_cllc_transformer_modA=global, ucs1_modA=global
  wires:
  i2_cllc_transformer/1 -> [i2_cllc_transformer_modA]
  u2_cllc_transformer/1 -> [u2_cllc_transformer_modA]
  u1_cllc_transformer/1 -> [u1_cllc_transformer_modA]
  i1_cllc_transformer/1 -> [i1_cllc_transformer_modA]
  single_phase_transformer/1 -> [single_phase_transformer_data_modA], single_phase_transformer - scope/1
  ucs/1 -> [ucs1_modA]
  [u1_cllc_transformer_modA] -> fsw/fres behaviour/1  "u1"
  [i1_cllc_transformer_modA] -> fsw/fres behaviour/2  "i1"
  [ucs1_modA] -> fsw/fres behaviour/3  "ucs1"
  [u2_cllc_transformer_modA] -> fsw/fres behaviour/4  "u2"
  connections:
  Current Sensor/RConn2 -- Voltage Sensor3/LConn1 -- u2(+)/RConn1
  Voltage Sensor3/RConn2 -- single_phase_transformer/RConn2 -- u2(-)/RConn1
  Current Sensor/RConn1 -- i2_cllc_transformer/LConn1
  Voltage Sensor3/RConn1 -- u2_cllc_transformer/LConn1
  u1(-)/RConn1 -- single_phase_transformer/LConn2 -- Voltage Sensor1/RConn2
  Current Sensor1/LConn1 -- Voltage Sensor1/LConn1 -- u1(+)/RConn1
  Voltage Sensor1/RConn1 -- u1_cllc_transformer/LConn1
  Current Sensor1/RConn1 -- i1_cllc_transformer/LConn1
  Current Sensor/LConn1 -- Capacitor1/RConn1
  single_phase_transformer/LConn1 -- Voltage Sensor2/LConn1 -- Capacitor/RConn1
  Capacitor/LConn1 -- Voltage Sensor2/RConn2 -- Current Sensor1/RConn2
  single_phase_transformer/RConn1 -- Capacitor1/LConn1
  ucs/LConn1 -- Voltage Sensor2/RConn1

== system sst_cllc_ttype_inv/dcdc_cllc_modA/dcdc_with_galvanic_isolation/full-bridge_1 ==
  gate_commands : Inport
  full-bridge_ideal_switch_based : Subsystem  Commented=on
  full-bridge_mosfet_based_with_thermal_model : Subsystem  Commented=on
  full-bridge_mosfet_based_with_thermal_model_zvs : Subsystem
  uac_1(+) : PMIOPort  Side=Left
  uac_1(-) : PMIOPort  Port=2  Side=Left
  Udc(+) : PMIOPort  Port=3  Side=Right
  Udc(-) : PMIOPort  Port=4  Side=Right
  wires:
  gate_commands/1 -> full-bridge_mosfet_based_with_thermal_model_zvs/1(gate_commands), full-bridge_ideal_switch_based/1(gate_commands), full-bridge_mosfet_based_with_thermal_model/1(gate_commands)
  connections:
  full-bridge_mosfet_based_with_thermal_model_zvs/LConn1 -- Udc(+)/RConn1 -- full-bridge_mosfet_based_with_thermal_model/LConn1 -- full-bridge_ideal_switch_based/LConn1
  full-bridge_mosfet_based_with_thermal_model_zvs/RConn1 -- full-bridge_mosfet_based_with_thermal_model/RConn1 -- full-bridge_ideal_switch_based/RConn1 -- uac_1(+)/RConn1
  full-bridge_mosfet_based_with_thermal_model_zvs/LConn2 -- Udc(-)/RConn1 -- full-bridge_ideal_switch_based/LConn2 -- full-bridge_mosfet_based_with_thermal_model/LConn2
  full-bridge_mosfet_based_with_thermal_model_zvs/RConn2 -- full-bridge_mosfet_based_with_thermal_model/RConn2 -- full-bridge_ideal_switch_based/RConn2 -- uac_1(-)/RConn1

== system sst_cllc_ttype_inv/dcdc_cllc_modA/dcdc_with_galvanic_isolation/full-bridge_2 ==
  gate_commands : Inport
  full-bridge_ideal_switch_based : Subsystem  Commented=on
  full-bridge_mosfet_based_with_thermal_model : Subsystem  Commented=on
  full-bridge_mosfet_based_with_thermal_model_zvs : Subsystem
  uac_1(+) : PMIOPort  Side=Left
  uac_1(-) : PMIOPort  Port=2  Side=Left
  Udc(+) : PMIOPort  Port=3  Side=Right
  Udc(-) : PMIOPort  Port=4  Side=Right
  wires:
  gate_commands/1 -> full-bridge_mosfet_based_with_thermal_model_zvs/1(gate_commands), full-bridge_ideal_switch_based/1(gate_commands), full-bridge_mosfet_based_with_thermal_model/1(gate_commands)
  connections:
  full-bridge_mosfet_based_with_thermal_model/LConn1 -- full-bridge_mosfet_based_with_thermal_model_zvs/LConn1 -- Udc(+)/RConn1 -- full-bridge_ideal_switch_based/LConn1
  full-bridge_mosfet_based_with_thermal_model/RConn1 -- full-bridge_mosfet_based_with_thermal_model_zvs/RConn1 -- full-bridge_ideal_switch_based/RConn1 -- uac_1(+)/RConn1
  full-bridge_mosfet_based_with_thermal_model_zvs/LConn2 -- full-bridge_mosfet_based_with_thermal_model/LConn2 -- Udc(-)/RConn1 -- full-bridge_ideal_switch_based/LConn2
  full-bridge_mosfet_based_with_thermal_model/RConn2 -- full-bridge_mosfet_based_with_thermal_model_zvs/RConn2 -- uac_1(-)/RConn1 -- full-bridge_ideal_switch_based/RConn2

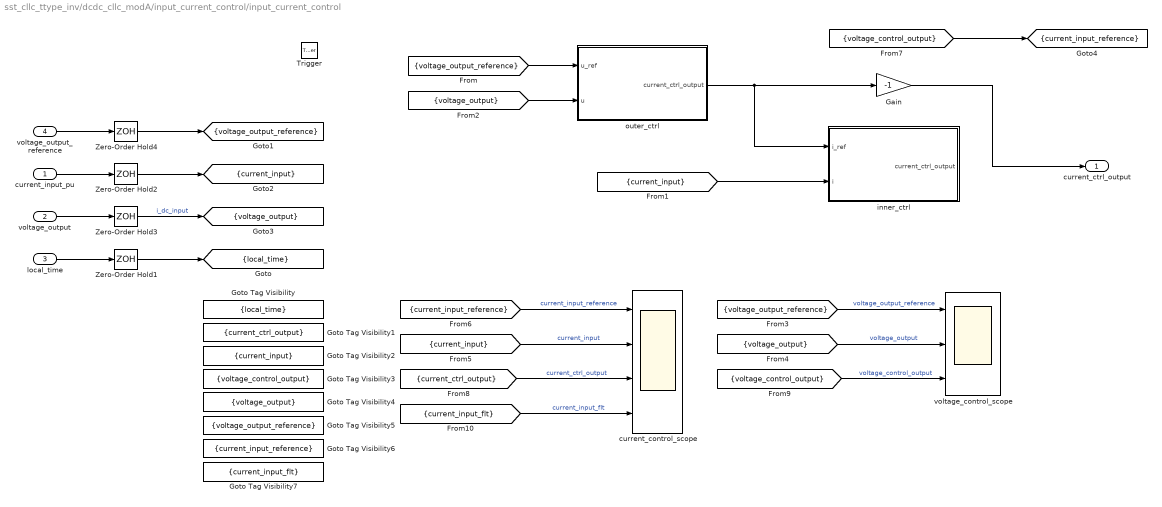
== system sst_cllc_ttype_inv/dcdc_cllc_modA/input_current_control/input_current_control ==
  current_input_pu : Inport
  voltage_output : Inport  Port=2
  local_time : Inport  Port=3
  voltage_output_reference : Inport  Port=4
  Trigger : TriggerPort  VariantControl=(inherit)  PortDimensions=1
  Gain : Gain  Gain=-1
  Goto Tag Visibility : GotoTagVisibility  GotoTag=local_time
  Goto Tag Visibility1 : GotoTagVisibility  GotoTag=current_ctrl_output
  Goto Tag Visibility2 : GotoTagVisibility  GotoTag=current_input
  Goto Tag Visibility3 : GotoTagVisibility  GotoTag=voltage_control_output
  Goto Tag Visibility4 : GotoTagVisibility  GotoTag=voltage_output
  Goto Tag Visibility5 : GotoTagVisibility  GotoTag=voltage_output_reference
  Goto Tag Visibility6 : GotoTagVisibility  GotoTag=current_input_reference
  Goto Tag Visibility7 : GotoTagVisibility  GotoTag=current_input_flt
  Zero-Order Hold{1..4} (4 alike) : ZeroOrderHold  SampleTime=-1
  current_control_scope : Scope  NumInputPorts=4
      settings: ActiveDisplayYMinimum=-1.72894287109375  ActiveDisplayYMaximum=5.56048583984375  DataLoggingVariableName=ScopeData12
  inner_ctrl : Subsystem
  outer_ctrl : Subsystem
  voltage_control_scope : Scope  NumInputPorts=3
      settings: ActiveDisplayYMinimum=-1.36859130859375  ActiveDisplayYMaximum=2.31732177734375  DataLoggingVariableName=ScopeData7
  current_ctrl_output : Outport
  tag scope: current_input=scoped, current_input_reference=scoped, local_time=scoped, voltage_output=scoped, voltage_output_reference=scoped
  wires:
  current_input_pu/1 -> Zero-Order Hold2/1
  local_time/1 -> Zero-Order Hold1/1
  voltage_output/1 -> Zero-Order Hold3/1
  Zero-Order Hold1/1 -> [local_time]
  voltage_output_reference/1 -> Zero-Order Hold4/1
  Zero-Order Hold4/1 -> [voltage_output_reference]
  Zero-Order Hold2/1 -> [current_input]
  Zero-Order Hold3/1 -> [voltage_output]  "i_dc_input"
  [voltage_output_reference] -> outer_ctrl/1(u_ref)
  outer_ctrl/1(current_ctrl_output) -> inner_ctrl/1(i_ref), Gain/1
  [current_input] -> inner_ctrl/2(i)
  [voltage_output] -> outer_ctrl/2(u)
  [current_input] -> current_control_scope/2  "current_input"
  [current_input_reference] -> current_control_scope/1  "current_input_reference"
  [voltage_control_output] -> [current_input_reference]
  [current_ctrl_output] -> current_control_scope/3  "current_ctrl_output"
  [voltage_output_reference] -> voltage_control_scope/1  "voltage_output_reference"
  [voltage_output] -> voltage_control_scope/2  "voltage_output"
  [voltage_control_output] -> voltage_control_scope/3  "voltage_control_output"
  [current_input_flt] -> current_control_scope/4  "current_input_flt"
  Gain/1 -> current_ctrl_output/1

== system sst_cllc_ttype_inv/dcdc_cllc_modA/input_current_control/modulator ==
  phase_displacement : Inport
  Constant1 : Constant  Value=0.5
  Constant2 : Constant  Value=0.5
  dab_single_phase_pwm_modulator : dab_single_phase_pwm_modulator/dab_single_phase_pwm_modulator  fPWM_DAB=glb_time.fPWM_CLLC  m_up=1  m_low=0  dead_time_DAB=glb_time.dead_time_CLLC  pos_cmd_gate=18  neg_cmd_gate=-3  polarity=-1  tc=glb_time.tc  max_phase_displacement=pi/2  trgo_double_update=glb_time.TRGO_CLLC_double_update
  gate_cmds : Outport
  tag scope: TRGO_cllc_modA=global
  wires:
  dab_single_phase_pwm_modulator/2 -> gate_cmds/1
  Constant2/1 -> dab_single_phase_pwm_modulator/3
  dab_single_phase_pwm_modulator/1 -> [TRGO_cllc_modA]
  Constant1/1 -> dab_single_phase_pwm_modulator/2
  [time_cllc_module_A] -> dab_single_phase_pwm_modulator/1
  phase_displacement/1 -> dab_single_phase_pwm_modulator/4

== system sst_cllc_ttype_inv/dcdc_cllc_modA/input_current_control/normalization ==
  in : Inport
  1/Ti3 : Gain  Gain=1/hwdata.cllc.idc1_bez  OutDataTypeStr=double  SaturateOnIntegerOverflow=on  ParamDataTypeStr=Inherit: Same as input
  Quantizer : Quantizer  QuantizationInterval=adc12_quantization
  out_pu : Outport
  wires:
  in/1 -> 1/Ti3/1
  1/Ti3/1 -> Quantizer/1
  Quantizer/1 -> out_pu/1

== system sst_cllc_ttype_inv/dcdc_cllc_modA/input_current_control/normalization1 ==
  in : Inport
  1/Ti3 : Gain  Gain=1/hwdata.cllc.udc2_bez  OutDataTypeStr=double  SaturateOnIntegerOverflow=on  ParamDataTypeStr=Inherit: Same as input
  Quantizer : Quantizer  QuantizationInterval=adc12_quantization
  out_pu : Outport
  wires:
  1/Ti3/1 -> Quantizer/1
  in/1 -> 1/Ti3/1
  Quantizer/1 -> out_pu/1

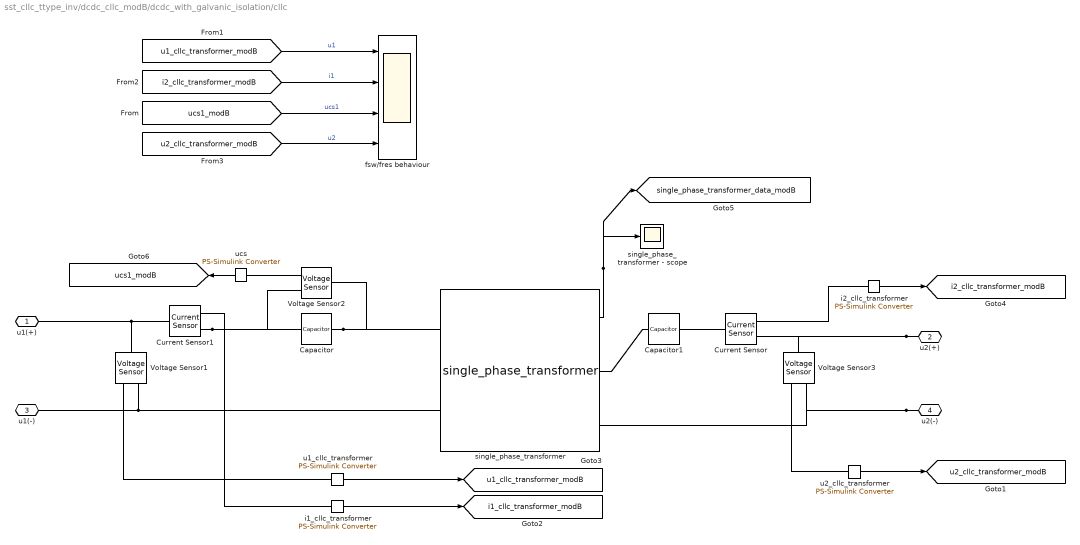
== system sst_cllc_ttype_inv/dcdc_cllc_modB/dcdc_with_galvanic_isolation/cllc ==
  Capacitor : fl_lib/Electrical/Electrical Elements/Capacitor  c=hwdata.cllc.Cs1 F  r=1e-6 Ohm  g=0 1/Ohm  i_specify=off  i_priority=None  i=0 A  i_nominal_specify=off  i_nominal_value=1  i_nominal_unit=A  v_specify=off  v_priority=None  v=0 V  v_nominal_specify=off  v_nominal_value=1  v_nominal_unit=V  vc_specify=off  vc_priority=High  vc=0 V  vc_nominal_specify=off  vc_nominal_value=1  vc_nominal_unit=V
  Capacitor1 : fl_lib/Electrical/Electrical Elements/Capacitor  c=hwdata.cllc.Cs2 F  r=1e-6 Ohm  g=0 1/Ohm  i_specify=off  i_priority=None  i=0 A  i_nominal_specify=off  i_nominal_value=1  i_nominal_unit=A  v_specify=off  v_priority=None  v=0 V  v_nominal_specify=off  v_nominal_value=1  v_nominal_unit=V  vc_specify=off  vc_priority=High  vc=0 V  vc_nominal_specify=off  vc_nominal_value=1  vc_nominal_unit=V
  Current Sensor : fl_lib/Electrical/Electrical Sensors/Current Sensor
  Current Sensor1 : fl_lib/Electrical/Electrical Sensors/Current Sensor
  Voltage Sensor1 : fl_lib/Electrical/Electrical Sensors/Voltage Sensor
  Voltage Sensor2 : fl_lib/Electrical/Electrical Sensors/Voltage Sensor
  Voltage Sensor3 : fl_lib/Electrical/Electrical Sensors/Voltage Sensor
  fsw/fres behaviour : Scope  NumInputPorts=4
      settings: ActiveDisplayYMinimum=-4267.1609835025592  ActiveDisplayYMaximum=3383.5844318464588  DataLoggingVariableName=ScopeData14
  i1_cllc_transformer : nesl_utility/PS-Simulink Converter  PhysicalDomain=network_engine_domain  SubClassName=ps_output  LeftPortType=input  RightPortType=output  PseudoPeriodic=off  Frequencies=[]  VectorFormat=1-D array  Unit=A  AffineConversion=off
  i2_cllc_transformer : nesl_utility/PS-Simulink Converter  PhysicalDomain=network_engine_domain  SubClassName=ps_output  LeftPortType=input  RightPortType=output  PseudoPeriodic=off  Frequencies=[]  VectorFormat=1-D array  Unit=A  AffineConversion=off
  single_phase_transformer : single_phase_transformer/single_phase_transformer  lm_trafo=hwdata.cllc.Lm  m1=hwdata.cllc.n1  m2=hwdata.cllc.n2  rd1_trafo=hwdata.cllc.Rs1  rd2_trafo=hwdata.cllc.Rs2  ld1_trafo=hwdata.cllc.Ld1  ld2_trafo=hwdata.cllc.Ld2  rfe_trafo=hwdata.cllc.Rfe  length_core=hwdata.cllc.core_length  mu0=1.256637e-6  mur=hwdata.cllc.core_mur
  single_phase_transformer - scope : Scope
      settings: ActiveDisplayYMinimum=-6684.1656967268027  ActiveDisplayYMaximum=6541.9063556817082  DataLoggingVariableName=ScopeData21
  u1_cllc_transformer : nesl_utility/PS-Simulink Converter  PhysicalDomain=network_engine_domain  SubClassName=ps_output  LeftPortType=input  RightPortType=output  PseudoPeriodic=off  Frequencies=[]  VectorFormat=1-D array  Unit=V  AffineConversion=on
  u2_cllc_transformer : nesl_utility/PS-Simulink Converter  PhysicalDomain=network_engine_domain  SubClassName=ps_output  LeftPortType=input  RightPortType=output  PseudoPeriodic=off  Frequencies=[]  VectorFormat=1-D array  Unit=V  AffineConversion=on
  ucs : nesl_utility/PS-Simulink Converter  PhysicalDomain=network_engine_domain  SubClassName=ps_output  LeftPortType=input  RightPortType=output  PseudoPeriodic=off  Frequencies=[]  VectorFormat=1-D array  Unit=V  AffineConversion=on
  u1(+) : PMIOPort  Side=Left
  u2(+) : PMIOPort  Port=2  Side=Right
  u1(-) : PMIOPort  Port=3  Side=Left
  u2(-) : PMIOPort  Port=4  Side=Right
  tag scope: i1_cllc_transformer_modB=global, i2_cllc_transformer_modB=global, single_phase_transformer_data_modB=global, u1_cllc_transformer_modB=global, u2_cllc_transformer_modB=global, ucs1_modB=global
  wires:
  [u2_cllc_transformer_modB] -> fsw/fres behaviour/4  "u2"
  [ucs1_modB] -> fsw/fres behaviour/3  "ucs1"
  [i2_cllc_transformer_modB] -> fsw/fres behaviour/2  "i1"
  [u1_cllc_transformer_modB] -> fsw/fres behaviour/1  "u1"
  ucs/1 -> [ucs1_modB]
  single_phase_transformer/1 -> single_phase_transformer - scope/1, [single_phase_transformer_data_modB]
  i1_cllc_transformer/1 -> [i1_cllc_transformer_modB]
  u1_cllc_transformer/1 -> [u1_cllc_transformer_modB]
  u2_cllc_transformer/1 -> [u2_cllc_transformer_modB]
  i2_cllc_transformer/1 -> [i2_cllc_transformer_modB]
  connections:
  ucs/LConn1 -- Voltage Sensor2/RConn1
  single_phase_transformer/RConn1 -- Capacitor1/LConn1
  Current Sensor1/RConn2 -- Voltage Sensor2/RConn2 -- Capacitor/LConn1
  Capacitor/RConn1 -- Voltage Sensor2/LConn1 -- single_phase_transformer/LConn1
  Current Sensor/LConn1 -- Capacitor1/RConn1
  Current Sensor1/RConn1 -- i1_cllc_transformer/LConn1
  Voltage Sensor1/RConn1 -- u1_cllc_transformer/LConn1
  u1(+)/RConn1 -- Voltage Sensor1/LConn1 -- Current Sensor1/LConn1
  Voltage Sensor1/RConn2 -- single_phase_transformer/LConn2 -- u1(-)/RConn1
  Voltage Sensor3/RConn1 -- u2_cllc_transformer/LConn1
  Current Sensor/RConn1 -- i2_cllc_transformer/LConn1
  u2(-)/RConn1 -- single_phase_transformer/RConn2 -- Voltage Sensor3/RConn2
  u2(+)/RConn1 -- Voltage Sensor3/LConn1 -- Current Sensor/RConn2

== system sst_cllc_ttype_inv/dcdc_cllc_modB/dcdc_with_galvanic_isolation/full-bridge_1 ==
  gate_commands : Inport
  full-bridge_ideal_switch_based : Subsystem
  full-bridge_mosfet_based_with_thermal_model : Subsystem  Commented=on
  full-bridge_mosfet_based_with_thermal_model_zvs : Subsystem  Commented=on
  uac_1(+) : PMIOPort  Side=Left
  uac_1(-) : PMIOPort  Port=2  Side=Left
  Udc(+) : PMIOPort  Port=3  Side=Right
  Udc(-) : PMIOPort  Port=4  Side=Right
  wires:
  gate_commands/1 -> full-bridge_mosfet_based_with_thermal_model/1(gate_commands), full-bridge_ideal_switch_based/1(gate_commands), full-bridge_mosfet_based_with_thermal_model_zvs/1(gate_commands)
  connections:
  uac_1(-)/RConn1 -- full-bridge_ideal_switch_based/RConn2 -- full-bridge_mosfet_based_with_thermal_model/RConn2 -- full-bridge_mosfet_based_with_thermal_model_zvs/RConn2
  full-bridge_mosfet_based_with_thermal_model/LConn2 -- full-bridge_ideal_switch_based/LConn2 -- Udc(-)/RConn1 -- full-bridge_mosfet_based_with_thermal_model_zvs/LConn2
  uac_1(+)/RConn1 -- full-bridge_ideal_switch_based/RConn1 -- full-bridge_mosfet_based_with_thermal_model/RConn1 -- full-bridge_mosfet_based_with_thermal_model_zvs/RConn1
  full-bridge_ideal_switch_based/LConn1 -- full-bridge_mosfet_based_with_thermal_model/LConn1 -- Udc(+)/RConn1 -- full-bridge_mosfet_based_with_thermal_model_zvs/LConn1

== system sst_cllc_ttype_inv/dcdc_cllc_modB/dcdc_with_galvanic_isolation/full-bridge_2 ==
  gate_commands : Inport
  full-bridge_ideal_switch_based : Subsystem
  full-bridge_mosfet_based_with_thermal_model : Subsystem  Commented=on
  full-bridge_mosfet_based_with_thermal_model_zvs : Subsystem  Commented=on
  uac_1(+) : PMIOPort  Side=Left
  uac_1(-) : PMIOPort  Port=2  Side=Left
  Udc(+) : PMIOPort  Port=3  Side=Right
  Udc(-) : PMIOPort  Port=4  Side=Right
  wires:
  gate_commands/1 -> full-bridge_mosfet_based_with_thermal_model/1(gate_commands), full-bridge_ideal_switch_based/1(gate_commands), full-bridge_mosfet_based_with_thermal_model_zvs/1(gate_commands)
  connections:
  full-bridge_ideal_switch_based/RConn2 -- uac_1(-)/RConn1 -- full-bridge_mosfet_based_with_thermal_model_zvs/RConn2 -- full-bridge_mosfet_based_with_thermal_model/RConn2
  full-bridge_ideal_switch_based/LConn2 -- Udc(-)/RConn1 -- full-bridge_mosfet_based_with_thermal_model/LConn2 -- full-bridge_mosfet_based_with_thermal_model_zvs/LConn2
  uac_1(+)/RConn1 -- full-bridge_ideal_switch_based/RConn1 -- full-bridge_mosfet_based_with_thermal_model_zvs/RConn1 -- full-bridge_mosfet_based_with_thermal_model/RConn1
  full-bridge_ideal_switch_based/LConn1 -- Udc(+)/RConn1 -- full-bridge_mosfet_based_with_thermal_model_zvs/LConn1 -- full-bridge_mosfet_based_with_thermal_model/LConn1
